simulink model "model_mux"  (R2023a)
settings: Solver=VariableStepAuto  StartTime=0.0  StopTime=10.0  RelTol=1e-3
settings Model: Creator=serviceadmin  LastModifiedBy=serviceadmin

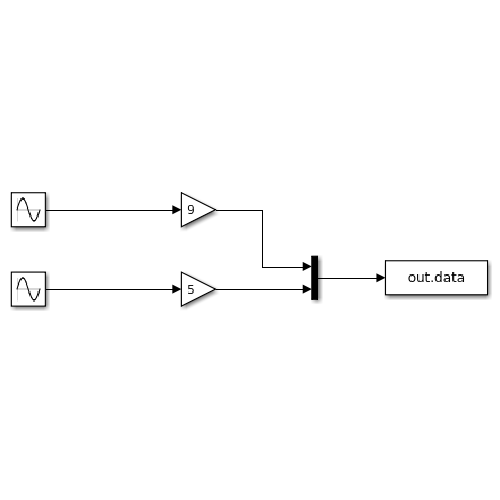
[thumbnail: Simulink's stored preview of the top-level diagram]
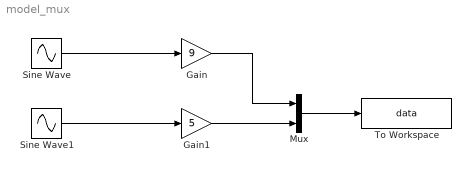
== system model_mux ==
  Gain : Gain  Gain=9
  Gain1 : Gain  Gain=5
  Mux : Mux  Inputs=2
  Sine Wave : Sin  SampleTime=0
  Sine Wave1 : Sin  SampleTime=0
  To Workspace : ToWorkspace  VariableName=data  SampleTime=-1
      settings: Save2DSignal=2-D array (concatenate along first dimension)
  wires:
  Sine Wave/1 -> Gain/1
  Gain/1 -> Mux/1
  Sine Wave1/1 -> Gain1/1
  Gain1/1 -> Mux/2
  Mux/1 -> To Workspace/1
